simulink model "Generator"  (R2024b)
settings: Solver=VariableStepAuto  StartTime=0.0  StopTime=10e-3  RelTol=1e-3
libraries: dspsrcs4 x3, commchan3 x1, dspvision x1
settings Model: Creator=mykola  LastModifiedBy=mykola

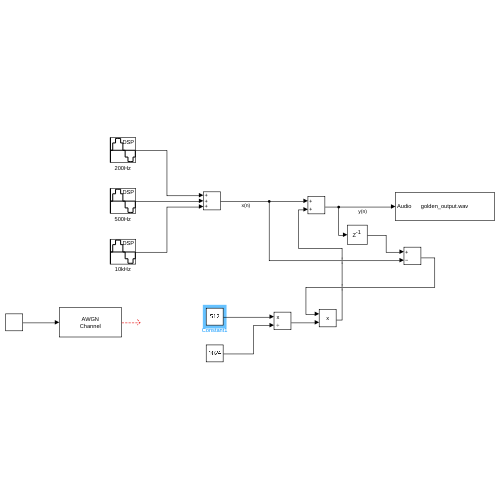
[thumbnail: Simulink's stored preview of the top-level diagram]
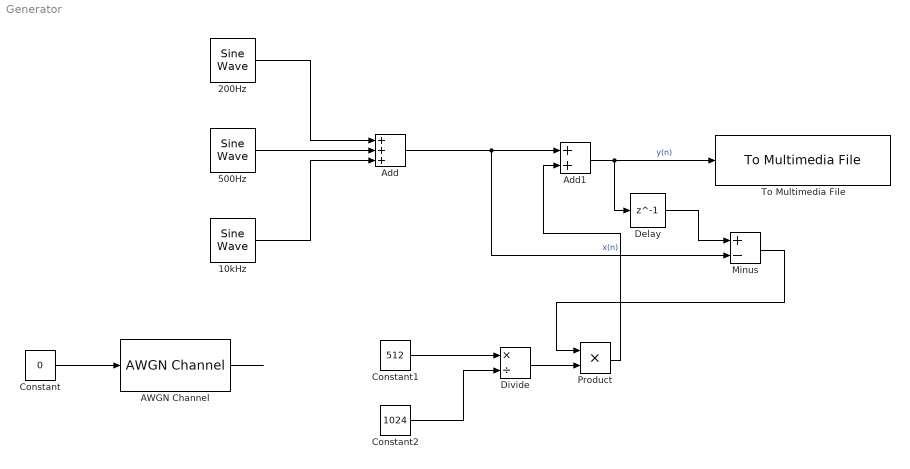
== system Generator ==
  10kHz : dspsrcs4/Sine Wave  Amplitude=0.3  Frequency=10e3  Phase=0  SampleMode=Discrete  OutComplex=Real  CompMethod=Trigonometric fcn  TableSize=Speed  SampleTime=1/44100  SamplesPerFrame=1  ResetState=Restart at time zero  OutputFrames=off  dataType=double  wordLen=16  udDataType=sfix(16)  fracBitsMode=Best precision  numFracBits=15  OutDataTypeStr=double  LastOutDataTypeStr=double
  200Hz : dspsrcs4/Sine Wave  Amplitude=0.3  Frequency=200  Phase=0  SampleMode=Discrete  OutComplex=Real  CompMethod=Trigonometric fcn  TableSize=Speed  SampleTime=1/44100  SamplesPerFrame=1  ResetState=Restart at time zero  OutputFrames=off  dataType=double  wordLen=16  udDataType=sfix(16)  fracBitsMode=Best precision  numFracBits=15  OutDataTypeStr=double  LastOutDataTypeStr=double
  500Hz : dspsrcs4/Sine Wave  Amplitude=0.3  Frequency=500  Phase=0  SampleMode=Discrete  OutComplex=Real  CompMethod=Trigonometric fcn  TableSize=Speed  SampleTime=1/44100  SamplesPerFrame=1  ResetState=Restart at time zero  OutputFrames=off  dataType=double  wordLen=16  udDataType=sfix(16)  fracBitsMode=Best precision  numFracBits=15  OutDataTypeStr=double  LastOutDataTypeStr=double
  AWGN Channel : commchan3/AWGN Channel  LegacyMode=off  NoiseMethod="Signal to noise ratio  (SNR)"  noiseMode="Signal to noise ratio  (SNR)"  EbNo=10  EsNo=10  SNR=0  BitsPerSymbol=1  SignalPower=1  SamplesPerSymbol=1  SymbolPeriod=1  VarianceSource=Parameter  Variance=1  RandomStream=Global stream  Seed=67  SimulateUsing=Code generation
  Add : Sum  Inputs=+++
  Add1 : Sum
  Constant : Constant  Value=0  SampleTime=1/44100
  Constant1 : Constant  Value=512
  Constant2 : Constant  Value=1024
  Delay : Delay  DelayLength=1
  Divide : Product  Inputs=*/
  Minus : Sum  Inputs=+-
  Product : Product
  To Multimedia File : dspvision/To Multimedia File  outputFilename=golden_output.wav  streamSelection=Audio only  videoCompressor=None (uncompressed)  audioCompressor=None (uncompressed)  imagePorts=One multidimensional signal  fileType=WAV  audioDatatype=16-bit integer  fourcc=RGB  audioBitRate=128  audioQuality=75  videoQuality=75  mj2000CompFactor=10
      settings: LibrarySourceBlock=dspsnks4/To Multimedia File
  wires:
  AWGN Channel/1 -> ?
  Constant/1 -> AWGN Channel/1
  200Hz/1 -> Add/1
  500Hz/1 -> Add/2
  10kHz/1 -> Add/3
  Add/1 -> Minus/2, Add1/1  "x(n)"
  Constant1/1 -> Divide/1
  Constant2/1 -> Divide/2
  Add1/1 -> Delay/1, To Multimedia File/1  "y(n)"
  Divide/1 -> Product/2
  Delay/1 -> Minus/1
  Minus/1 -> Product/1
  Product/1 -> Add1/2
